simulink model "dspsdadc"  (R2017b)
settings: Solver=ode5  StartTime=0.0  StopTime=1  MaxStep=1/512000  RelTol=1e-3  AbsTol=1e-6
model workspace (MAT data in the model file):
  Fs = 512000
  fir_fc = 0.258
  fir_order = 511
libraries: dspmlti4 x6, dsparch4 x1, simulink x1, dspmisc x1, dspstat3 x1
settings Model: ExtModeTrigMode=oneshot  ExtModeArmWhenConnect=off  ExtModeAutoUpdateStatusClock=off  Creator=The MathWorks, Inc.  LastModifiedBy=Niko
settings DataIOCC: SaveFormat=Array  SaveOutput=off  SaveTime=off  SignalLoggingName=logsOut
settings OptimizationCC: BlockReduction=off  BooleanDataType=off  ExpressionDepthLimit=2147483647  RollThreshold=2  InitFltsAndDblsToZero=on  EfficientMapNaN2IntZero=off  LifeSpan=inf  SimCompilerOptimization=on
settings DebuggingCC: SaveWithParameterizedLinksMsg=none  UnderspecifiedInitializationDetection=Classic  MergeDetectMultiDrivingBlocksExec=none  SignalResolutionControl=TryResolveAllWithWarning  MultiTaskDSMMsg=warning  MultiTaskCondExecSysMsg=none  IntegerOverflowMsg=none  FcnCallInpInsideContextMsg=warning  AllowSymbolicDim=off  StateNameClashWarn=warning  SFUnexpectedBacktrackingDiag=warning  SFNoUnconditionalDefaultTransitionDiag=warning  SFExecutionAtInitializationDiag=none  IntegerSaturationMsg=none
settings HardwareCC: ProdBitPerPointer=32  ProdBitPerSizeT=32  ProdBitPerPtrDiffT=32  ProdLargestAtomicFloat=None  ProdIntDivRoundTo=Undefined  ProdEndianess=Unspecified  ProdWordSize=32  ProdHWDeviceType=32-bit Generic  TargetUnknown=on
settings ModelReferenceCC: PropagateSignalLabelsOutOfModel=off
settings CodeAppCC: StateflowObjectComments=on
settings GRTTargetCC: TargetFcnLib=ansi_tfl_tmw.mat  TargetLangStandard=C89/C90 (ANSI)  GeneratePreprocessorConditionals=Disable all  CombineOutputUpdateFcns=off  GRTInterface=on
settings ConfigComp: CovMetricSettings=dw  CovHtmlReporting=on  CovSaveCumulativeToWorkspaceVar=on  CovSaveSingleToWorkspaceVar=on  CovExternalEMLEnable=off

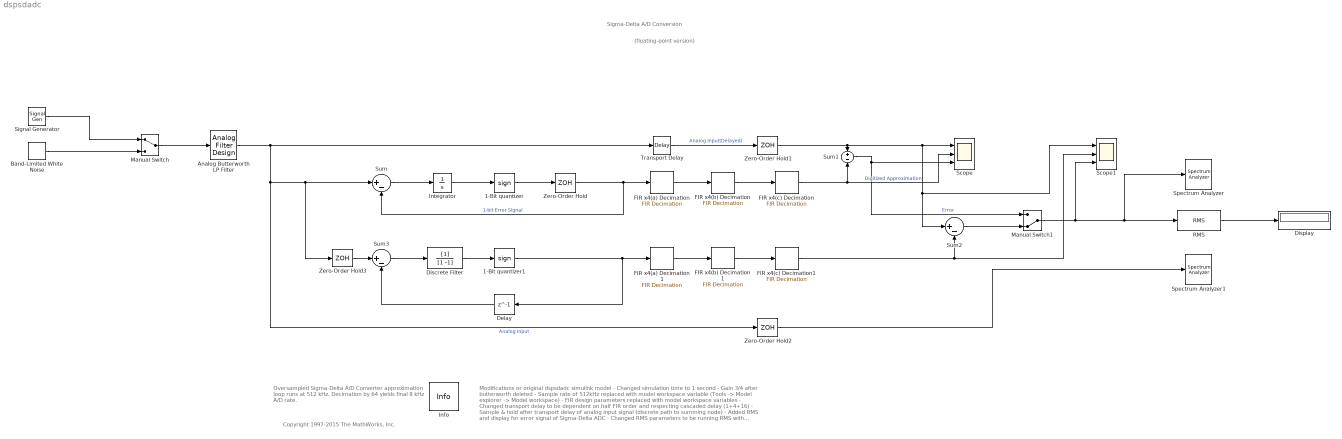
== system dspsdadc ==
  note: Modifications or original dspsdadc simulink model
      |
      | - Changed simulation time to 1 second
      | - Gain 3/4 after butterworth deleted
      | - Sample rate of 512kHz replaced with model workspace variable (Tools -> Model explorer -> Model workspace)
      | - FIR design parameters replaced with model workspace variables
      | - Changed transport delay to be dependent on half FIR order and respecting cascaded delay (1+4+16)
      | - Sample & hold after transport delay of analog input signal (discrete path to summing node)
      | - Added RMS and display for error signal of Sigma-Delta ADC
      | - Changed RMS parameters to be running RMS with sampled-based input -> Better averaging over time
      | - Added spectrum analyzer nodes for analog input signal and error signal
      | - FIR design parameters changed from default to:
      | - order: 511
      | - cutoff: 0.258
      | - Apply blackman window for FIR filters
      | - Changed ampitude and frequency of signal generator
      | - Amplitude: 0.6
      | - Frequency: 200
      | - Changed characteristics of butterworth LP filter
      | - Order: 80
      | - Cutoff: 3800Hz -> 4000Hz band-limited signal (because final Fs will be 8kHz = 512kHz/64)
      | - Added option to toggle input source between signal generator and white noise generator with following characteristics:
      | - Amplitude: 0.000005
      | - Sample time: 1/Fs
  note: Oversampled Sigma-Delta A/D Converter
      | approximation loop runs at 512 kHz.
      | Decimation by 64 yields final 8 kHz A/D rate.
  note: Copyright 1997-2015 The MathWorks, Inc.
  note: Sigma-Delta A/D Conversion
  note: (floating-point version)
  1-Bit quantizer : Signum
  1-Bit quantizer1 : Signum
  Analog Butterworth LP Filter : dsparch4/Analog Filter Design  method=Butterworth  filttype=Lowpass  N=80  Wlo=2*pi*3800  Whi=80  Rp=2  Rs=40
  Band-Limited White Noise : simulink/Sources/Band-Limited White Noise  Cov=[0.000005]  Ts=1/Fs  seed=[23341]
  Delay : Delay  DelayLength=1  InitialCondition=0
  Discrete Filter : DiscreteFilter  Denominator=[1 -1]
  Display : Display
  FIR x4(a) Decimation : dspmlti4/FIR Decimation  FilterSource=Dialog parameters  h=fir1(fir_order,fir_fc,window(@blackman,fir_order+1))  D=4  filtStruct=Direct form  FilterObject=Hm_firdecim  framing=Allow multirate processing  inputOffset=0  outputBufInitCond=0  roundingMode=Floor  overflowMode=off  firstCoeffDataTypeStr=Inherit: Same word length as input  firstCoeffMin=[]  firstCoeffMax=[]  firstCoeffLastDataTypeStr=Inherit: Same word length as input  accumDataTypeStr=Inherit: Same as product output  accumLastDataTypeStr=Inherit: Same as product output  outputMin=[]  outputMax=[]
  FIR x4(a) Decimation1 : dspmlti4/FIR Decimation  FilterSource=Dialog parameters  h=fir1(fir_order,fir_fc,window(@blackman,fir_order+1))  D=4  filtStruct=Direct form  FilterObject=Hm_firdecim  framing=Allow multirate processing  inputOffset=0  outputBufInitCond=0  roundingMode=Floor  overflowMode=off  firstCoeffDataTypeStr=Inherit: Same word length as input  firstCoeffMin=[]  firstCoeffMax=[]  firstCoeffLastDataTypeStr=Inherit: Same word length as input  accumDataTypeStr=Inherit: Same as product output  accumLastDataTypeStr=Inherit: Same as product output  outputMin=[]  outputMax=[]
  FIR x4(b) Decimation : dspmlti4/FIR Decimation  FilterSource=Dialog parameters  h=fir1(fir_order,fir_fc,window(@blackman,fir_order+1))  D=4  filtStruct=Direct form  FilterObject=Hm_firdecim  framing=Allow multirate processing  inputOffset=0  outputBufInitCond=0  roundingMode=Floor  overflowMode=off  firstCoeffDataTypeStr=Inherit: Same word length as input  firstCoeffMin=[]  firstCoeffMax=[]  firstCoeffLastDataTypeStr=Inherit: Same word length as input  accumDataTypeStr=Inherit: Same as product output  accumLastDataTypeStr=Inherit: Same as product output  outputMin=[]  outputMax=[]
  FIR x4(b) Decimation1 : dspmlti4/FIR Decimation  FilterSource=Dialog parameters  h=fir1(fir_order,fir_fc,window(@blackman,fir_order+1))  D=4  filtStruct=Direct form  FilterObject=Hm_firdecim  framing=Allow multirate processing  inputOffset=0  outputBufInitCond=0  roundingMode=Floor  overflowMode=off  firstCoeffDataTypeStr=Inherit: Same word length as input  firstCoeffMin=[]  firstCoeffMax=[]  firstCoeffLastDataTypeStr=Inherit: Same word length as input  accumDataTypeStr=Inherit: Same as product output  accumLastDataTypeStr=Inherit: Same as product output  outputMin=[]  outputMax=[]
  FIR x4(c) Decimation : dspmlti4/FIR Decimation  FilterSource=Dialog parameters  h=fir1(fir_order,fir_fc,window(@blackman,fir_order+1))  D=4  filtStruct=Direct form  FilterObject=Hm_firdecim  framing=Allow multirate processing  inputOffset=0  outputBufInitCond=0  roundingMode=Floor  overflowMode=off  firstCoeffDataTypeStr=Inherit: Same word length as input  firstCoeffMin=[]  firstCoeffMax=[]  firstCoeffLastDataTypeStr=Inherit: Same word length as input  accumDataTypeStr=Inherit: Same as product output  accumLastDataTypeStr=Inherit: Same as product output  outputMin=[]  outputMax=[]
  FIR x4(c) Decimation1 : dspmlti4/FIR Decimation  FilterSource=Dialog parameters  h=fir1(fir_order,fir_fc,window(@blackman,fir_order+1))  D=4  filtStruct=Direct form  FilterObject=Hm_firdecim  framing=Allow multirate processing  inputOffset=0  outputBufInitCond=0  roundingMode=Floor  overflowMode=off  firstCoeffDataTypeStr=Inherit: Same word length as input  firstCoeffMin=[]  firstCoeffMax=[]  firstCoeffLastDataTypeStr=Inherit: Same word length as input  accumDataTypeStr=Inherit: Same as product output  accumLastDataTypeStr=Inherit: Same as product output  outputMin=[]  outputMax=[]
  Info : dspmisc/Info  SystemSampleTime=-1
      settings: SourceProductName=DSP System Toolbox  SourceProductBaseCode=DS
  Integrator : Integrator
  Manual Switch : ManualSwitch
  Manual Switch1 : ManualSwitch  CurrentSetting=0
  RMS : dspstat3/RMS  run=on  directionMode=Each column  dimension=1  reset_popup=None
  Scope : Scope  NumInputPorts=3
  Scope1 : Scope  NumInputPorts=3
  Signal Generator : SignalGenerator  WaveForm=square  Amplitude=0.6  Frequency=200
  Spectrum Analyzer : SpectrumAnalyzer
  Spectrum Analyzer1 : SpectrumAnalyzer
  Sum : Sum  Inputs=|+-  SaturateOnIntegerOverflow=on  InputSameDT=on  OutDataTypeStr=Inherit: Same as first input
  Sum1 : Sum  Inputs=+-  SaturateOnIntegerOverflow=on  InputSameDT=on  OutDataTypeStr=Inherit: Same as first input
  Sum2 : Sum  Inputs=|+-  SaturateOnIntegerOverflow=on  InputSameDT=on  OutDataTypeStr=Inherit: Same as first input
  Sum3 : Sum  Inputs=|+-  SaturateOnIntegerOverflow=on  InputSameDT=on  OutDataTypeStr=Inherit: Same as first input
  Transport Delay : TransportDelay  DelayTime=(1+4+16)*(fir_order/2)/Fs
  Zero-Order Hold : ZeroOrderHold  SampleTime=1/Fs
  Zero-Order Hold1 : ZeroOrderHold  SampleTime=(4*4*4)/Fs %Reduced sampling rate due to oversampling factor
  Zero-Order Hold2 : ZeroOrderHold  SampleTime=(4*4*4)/Fs %Reduced sampling rate due to oversampling factor
  Zero-Order Hold3 : ZeroOrderHold  SampleTime=1/Fs
  wires:
  Zero-Order Hold/1 -> Sum/2, FIR x4(a) Decimation/1  "1-bit Error Signal"
  1-Bit quantizer/1 -> Zero-Order Hold/1
  Sum/1 -> Integrator/1
  Integrator/1 -> 1-Bit quantizer/1
  FIR x4(c) Decimation/1 -> Scope/2, Sum1/2  "Digitized Approximation"
  Analog Butterworth LP Filter/1 -> Transport Delay/1, Sum/1, Zero-Order Hold3/1, Zero-Order Hold2/1  "Analog Input"
  Signal Generator/1 -> Manual Switch/1
  FIR x4(a) Decimation/1 -> FIR x4(b) Decimation/1
  FIR x4(b) Decimation/1 -> FIR x4(c) Decimation/1
  Sum1/1 -> Manual Switch1/1, Scope/3  "Error"
  Transport Delay/1 -> Zero-Order Hold1/1  "Analog Input(Delayed)"
  Zero-Order Hold1/1 -> Sum2/1, Scope1/1, Scope/1, Sum1/1
  RMS/1 -> Display/1
  Zero-Order Hold2/1 -> Spectrum Analyzer1/1
  Manual Switch/1 -> Analog Butterworth LP Filter/1
  Band-Limited White Noise/1 -> Manual Switch/2
  Delay/1 -> Sum3/2
  Sum3/1 -> Discrete Filter/1
  Discrete Filter/1 -> 1-Bit quantizer1/1
  1-Bit quantizer1/1 -> Delay/1, FIR x4(a) Decimation1/1
  FIR x4(a) Decimation1/1 -> FIR x4(b) Decimation1/1
  FIR x4(b) Decimation1/1 -> FIR x4(c) Decimation1/1
  Zero-Order Hold3/1 -> Sum3/1
  FIR x4(c) Decimation1/1 -> Sum2/2, Scope1/2
  Manual Switch1/1 -> RMS/1, Spectrum Analyzer/1, Scope1/3
  Sum2/1 -> Manual Switch1/2
